simulink model "Cognata_Amp_Tobi_Split_Excel"  (R2020a)
settings: Solver=VariableStepAuto  StartTime=0.0  StopTime=inf  RelTol=1e-3
model workspace (MAT data in the model file):
  WinSize = Simulink.Parameter
  WinSize.Value = 16
  WinSize.DataType = 'double'
  WinSize.Dimensions = [1 1]
  fc_bandpass = Simulink.Parameter
  fc_bandpass.Value = [0.05 0.26]
  fc_bandpass.DataType = 'double'
  fc_bandpass.Dimensions = [1 2]
undefined symbols (not defined in the file or in its folder): A1, A138674, A91496, C1, currentCFG_Cognata_Amp_Tobi_split_UB, I1, J138674, O91496, UB, W1, W91496
libraries: gtecHighspeedLib x1, gUSBamplib x1
settings Model: Creator=LAB-OREN3  LastModifiedBy=LAB-OREN3

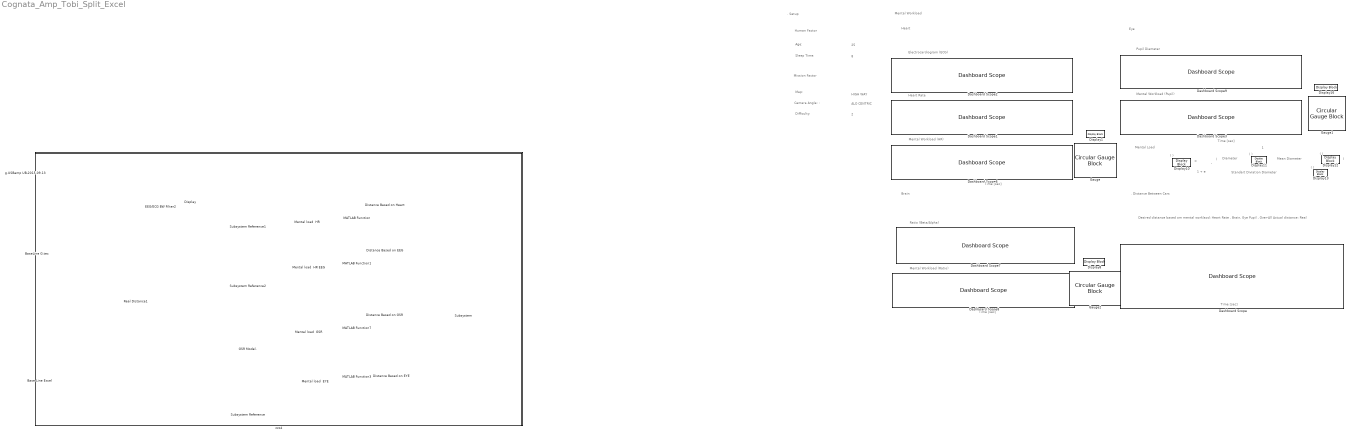
== system Cognata_Amp_Tobi_Split_Excel ==
  note: Mental Load
  note: Difficulty:
  note: Brain
  note: ( )
  note: ( )
  note: 1 + e
  note: . Setup
  note: Map:
  note: Diameter
  note: )
  note: Heart Rate
  note: Heart
  note: -
  note: ALO CENTRIC
  note: Time [sec]
  note: . Distance Between Cars
  note: Desired distance based om mental worklaod:
      | Heart Rate , Brain, Eye Pupil , Over-All
      |
      | Actual distance: Real
  note: HIGH WAY
  note: Sleep Time:
  note: 2
  note: Time [sec]
  note: Human Factor
  note: 1
  note: Electrocardiogram (ECG)
  note: Standart Diviation Diameter
  note: Mental Workload (HR)
  note: Ratio (Beta/Alpha)
  note: Time [sec]
  note: 25
  note: (
  note: 8
  note: Camera Angle: :
  note: Eye
  note: Mental Workload (Ratio)
  note: ( )
  note: =
  note: Pupil Diameter
  note: Mental Workload (Pupil)
  note: Time [sec]
  note: ( )
  note: Mission Factor
  note: Mean Diameter
  note: Mental Workload
  note: Age:
  Base Line Excel : FromSpreadsheet  FileName=C:\Users\LAB-OREN3\Downloads\1\Tobii Data of A2_535986_COMBINED_CUBE_DELAY_50_TTC_15 at (15;28;36).xlsx  SheetName=גיליון1  Range=A1:A138674,I1:J138674  SampleTime=0.001953125
  BaseLine G.tec : FromSpreadsheet  FileName=C:\Users\LAB-OREN3\Downloads\1\g.techAmp Data of A2_535986_COMBINED_CUBE_DELAY_50_TTC_15 at (15;28;36).xlsx  SheetName=גיליון1  Range=A1:A91496,C1:O91496,W1:W91496  SampleTime=0.001953125
  Dashboard Scope : DashboardScope  ShowInitialText=off  TimeSpan=10  Ymin=-1  Ymax=20  LegendPosition=Hide  ScaleAtStop=off
  Dashboard Scope1 : DashboardScope  TimeSpan=10  Ymin=0  Ymax=100  LegendPosition=Hide  ScaleAtStop=off
  Dashboard Scope2 : DashboardScope  TimeSpan=10  Ymin=-3000  Ymax=1000  LegendPosition=Hide  ScaleAtStop=off
  Dashboard Scope3 : DashboardScope  TimeSpan=10  Ymin=0  Ymax=1  LegendPosition=Hide  ScaleAtStop=off
  Dashboard Scope6 : DashboardScope  TimeSpan=10  Ymin=0  Ymax=1  LegendPosition=Hide  ScaleAtStop=off
  Dashboard Scope7 : DashboardScope  TimeSpan=10  Ymin=0  Ymax=0.5  LegendPosition=Hide  ScaleAtStop=off
  Dashboard Scope8 : DashboardScope  TimeSpan=10  Ymin=0  Ymax=1  LegendPosition=Hide  ScaleAtStop=off
  Dashboard Scope9 : DashboardScope  TimeSpan=10  Ymin=0  Ymax=5  LegendPosition=Hide  ScaleAtStop=off
  Display : Display
  Display{1,8,10..11,13,16} (6 alike) : DisplayBlock  LabelPosition=Hide  Format=bank  Transparency=1
  Display12 : DisplayBlock  LabelPosition=Hide  Format=bank  Transparency=1  Layout=Fill available space
  Distance Based on EEG : Display
  Distance Based on EYE : Display
  Distance Based on GSR : Display
  Distance Based on Heart : Display
  EEG/ECG BW Filter2 : gtecHighspeedLib/EEG//ECG BW Filter  Order=6  LowerFreq=0.1  UpperFreq=30  SampFreq=512
      settings: SourceProductName=g.HIsys Library
  GSR Model. : Subsystem
  Gauge : CircularGaugeBlock  LabelPosition=Hide  ScaleMax=1  TickInterval=0.2
  Gauge1 : CircularGaugeBlock  LabelPosition=Hide  ScaleMax=1  TickInterval=0.2
  Gauge2 : CircularGaugeBlock  LabelPosition=Hide  ScaleMax=1  TickInterval=0.2
  MATLAB Function : MATLAB Function  TreatAsAtomicUnit=on
  MATLAB Function1 : MATLAB Function  TreatAsAtomicUnit=on
  MATLAB Function3 : MATLAB Function  TreatAsAtomicUnit=on
  MATLAB Function7 : MATLAB Function  TreatAsAtomicUnit=on
  Mental load  EYE : MATLAB Function  TreatAsAtomicUnit=on
  Mental load  GSR : MATLAB Function  TreatAsAtomicUnit=on
  Mental load  HR : MATLAB Function  TreatAsAtomicUnit=on
  Mental load  HR EEG : MATLAB Function  TreatAsAtomicUnit=on
  Real Distance1 : MATLAB Function  TreatAsAtomicUnit=on
  Subsystem : Subsystem
  Subsystem Reference : Subsystem  ReferencedSubsystem=Pupil_Diameter_Model
  Subsystem Reference1 : Subsystem  ReferencedSubsystem=Heart_Rate_Model
  Subsystem Reference2 : Subsystem  ReferencedSubsystem=EEG_Ratio_Model
  g.USBamp UB-2015.09.13 : gUSBamplib/g.USBamp  cfg=currentCFG_Cognata_Amp_Tobi_split_UB-2015.09.13.cfg  snr=UB-2015.09.13
      settings: SourceProductName=g.USBamp
  zzz4 : Subsystem  TreatAsAtomicUnit=on
      settings: OpenFcn=% no-op
      mask Display: disp('')
  wires:
  Mental load  HR EEG/1(y) -> MATLAB Function1/1(u), Subsystem/2(Ratio)
  MATLAB Function/1(y) -> Distance Based on Heart/1
  MATLAB Function3/1(y) -> Distance Based on EYE/1
  Mental load  HR/1(y) -> MATLAB Function/1(u), Subsystem/1(HR)
  MATLAB Function1/1(y) -> Distance Based on EEG/1
  Mental load  EYE/1(y) -> MATLAB Function3/1(u), Subsystem/4(eye)
  Subsystem Reference2/1 -> Mental load  HR EEG/1(u)
  Base Line Excel/1 -> Subsystem Reference/1
  Base Line Excel/2 -> Subsystem Reference/2
  Subsystem Reference/1 -> Mental load  EYE/1(u)
  BaseLine G.tec/2 -> EEG/ECG BW Filter2/1, Subsystem Reference1/1
  Subsystem Reference1/2 -> Mental load  HR/1(u)
  BaseLine G.tec/3 -> Subsystem Reference2/1
  BaseLine G.tec/4 -> Subsystem Reference2/2
  BaseLine G.tec/5 -> Subsystem Reference2/3
  BaseLine G.tec/6 -> Subsystem Reference2/4
  BaseLine G.tec/7 -> Subsystem Reference2/5
  BaseLine G.tec/8 -> Subsystem Reference2/6
  BaseLine G.tec/9 -> Subsystem Reference2/7
  BaseLine G.tec/10 -> Subsystem Reference2/8
  BaseLine G.tec/11 -> Subsystem Reference2/9
  BaseLine G.tec/12 -> Subsystem Reference2/10
  BaseLine G.tec/13 -> Subsystem Reference2/11
  BaseLine G.tec/1 -> GSR Model./1(In1)
  Mental load  GSR/1(y) -> MATLAB Function7/1(u), Subsystem/3(GSR)
  MATLAB Function7/1(y) -> Distance Based on GSR/1
  GSR Model./1(GSR) -> Mental load  GSR/1(u)
  EEG/ECG BW Filter2/1 -> Display/1
  BaseLine G.tec/14 -> Real Distance1/1(u)
  Real Distance1/1(y) -> ?
  Subsystem/1(Avrage Mental Load) -> ?
  Subsystem Reference/2 -> ?
  Subsystem Reference/3 -> ?

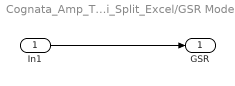
== system Cognata_Amp_Tobi_Split_Excel/GSR Model. ==
  In1 : Inport
  GSR : Outport
  wires:
  In1/1 -> GSR/1

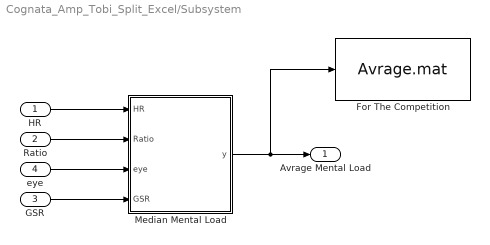
== system Cognata_Amp_Tobi_Split_Excel/Subsystem ==
  HR : Inport
  Ratio : Inport  Port=2
  GSR : Inport  Port=3
  eye : Inport  Port=4
  For The Competition : ToFile  Filename=Avrage.mat  MatrixName=Avrage
  Median Mental Load : MATLAB Function  TreatAsAtomicUnit=on
  Avrage Mental Load : Outport
  wires:
  GSR/1 -> Median Mental Load/4(GSR)
  Median Mental Load/1(y) -> For The Competition/1, Avrage Mental Load/1
  Ratio/1 -> Median Mental Load/2(Ratio)
  eye/1 -> Median Mental Load/3(eye)
  HR/1 -> Median Mental Load/1(HR)

== system Cognata_Amp_Tobi_Split_Excel/zzz4 ==

== matlab function Cognata_Amp_Tobi_Split_Excel/MATLAB Function ==
  data: u input; y output
function y = fcn(u)
%#codegen

y = (u*10)+10;

== matlab function Cognata_Amp_Tobi_Split_Excel/Real Distance1 ==
  data: u input; y output
function y = fcn(u)

y = u;

== matlab function Cognata_Amp_Tobi_Split_Excel/Mental load  HR ==
  data: u input; y output
function y = fcn(u)

y= probability_of_mental_load_HR(u);

end

== matlab function Cognata_Amp_Tobi_Split_Excel/Subsystem/Median Mental Load ==
  data: HR input; y output; Ratio input; eye input; GSR input
function y = fcn(HR, Ratio, eye, GSR)


    vac = [HR Ratio,eye,GSR];
    y = median(vac);

end

== matlab function Cognata_Amp_Tobi_Split_Excel/Mental load  HR EEG ==
  data: u input; y output
function y = fcn(u)

y= probability_of_metal_load_EEG(u);

end

== matlab function Cognata_Amp_Tobi_Split_Excel/MATLAB Function1 ==
  data: u input; y output
function y = fcn(u)
%#codegen

y = (u*10)+10;

== matlab function Cognata_Amp_Tobi_Split_Excel/Mental load  EYE ==
  data: u input; y output
function y = fcn( u)

y= probability_of_metal_load_EYE(u);

end

== matlab function Cognata_Amp_Tobi_Split_Excel/MATLAB Function3 ==
  data: u input; y output
function y = fcn(u)
%#codegen

y = (u*10)+10;

== matlab function Cognata_Amp_Tobi_Split_Excel/Mental load  GSR ==
  data: u input; y output
function y = fcn(u)

y= probability_of_metal_load_GSR(u);

end

== matlab function Cognata_Amp_Tobi_Split_Excel/MATLAB Function7 ==
  data: u input; y output
function y = fcn(u)
%#codegen

y = (u*10)+10;
